simulink model "threePhaseInverterOpenLoop"  (R2021a)
settings: Solver=VariableStepAuto  StartTime=0.0  StopTime=.18  RelTol=1e-3
libraries: spsIGBTDiodeLib x12, spsTHDLib x6, spsSeriesRLCBranchLib x6, spsVoltageMeasurementLib x6, spsDCVoltageSourceLib x4, spsGroundLib x4, spsTriangleGeneratorLib x2, spsCurrentMeasurementLib x2, spspowerguiLib x1
settings Model: Creator=User  LastModifiedBy=User
settings SolverCC: AlgebraicLoopSolver=TrustRegion
settings DebuggingCC: SFMachineParentedDataDiag=warning

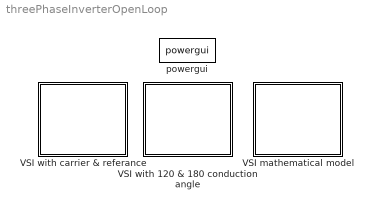
== system threePhaseInverterOpenLoop ==
  VSI mathematical model : Subsystem
  VSI with 120 & 180 conduction angle : Subsystem
  VSI with carrier & referance : Subsystem
  powergui : spspowerguiLib/powergui  Priority=1  SimulationMode=Continuous  SampleTime=50e-6  frequency=60  Iterations=50  frequencyindice=0  Pbase=100e6  ErrMax=1e-4  UnitsV=kV  UnitsW=MW  buscounter=0  FunctionMessages=off  echomessages=off  EnableUseOfTLC=off  CurrentSourceSwitches=off  DisableSnubberDevices=on  DisableRonSwitches=on  DisableVfSwitches=on  DisplayEquations=off  AutomaticDiscreteSolvers=off  SolverType=Tustin/Backward Euler (TBE)  Interpol=off  ExternalGateDelay=off  methode=off  Ts=100  x0status=blocks  SPID=on  SwTol=0  HookPort=off  NonlinearTolerance=1e-4  nMaxIteration=100  ContinueOnMaxIteration=off  RestoreLinks=warning  ResistiveCurrentMeasurement=off  Frange=[0:2:500]  Ylog=off  Xlog=on  ShowGrid=off  save=off  variable=ZData  structure=0  ZoomFFT=off  StartTime=0.0  cycles=1  DisplayStyle=1  fundamental=60  FreqAxis=off  MaxFrequency=1000  frequencyindicesteady=1  RmsSteady=1  display=off

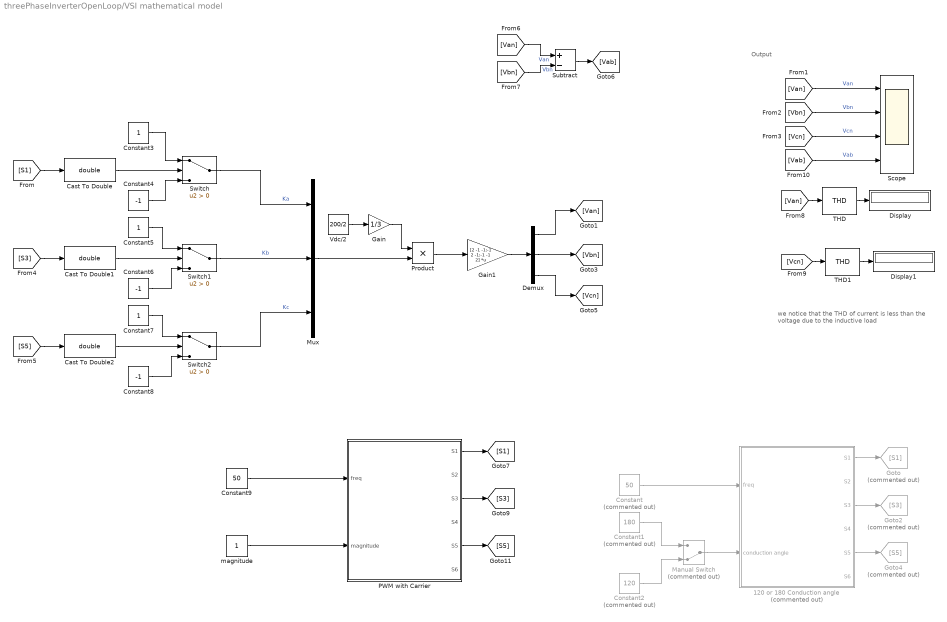
== system threePhaseInverterOpenLoop/VSI mathematical model ==
  note: we notice that the THD of current is less than the voltage due to the inductive load
  note: Output
  120 or 180 Conduction angle : Subsystem  Commented=on
  Cast To Double : DataTypeConversion  OutDataTypeStr=double
  Cast To Double1 : DataTypeConversion  OutDataTypeStr=double
  Cast To Double2 : DataTypeConversion  OutDataTypeStr=double
  Constant : Constant  Commented=on  Value=50
  Constant1 : Constant  Commented=on  Value=180
  Constant2 : Constant  Commented=on  Value=120
  Constant3 : Constant
  Constant4 : Constant  Value=-1
  Constant5 : Constant
  Constant6 : Constant  Value=-1
  Constant7 : Constant
  Constant8 : Constant  Value=-1
  Constant9 : Constant  Value=50
  Demux : Demux  Outputs=3
  Display : Display
  Display1 : Display
  Gain : Gain  Gain=1/3
  Gain1 : Gain  Gain=[2 -1 -1;-1 2 -1;-1 -1 2]  Multiplication=Matrix(K*u)
  Goto : Goto  Commented=on  GotoTag=S1
  Goto2 : Goto  Commented=on  GotoTag=S3
  Goto4 : Goto  Commented=on  GotoTag=S5
  Manual Switch : ManualSwitch  Commented=on  CurrentSetting=0
  Mux : Mux  Inputs=3
  PWM with Carrier : Subsystem
  Product : Product
  Scope : Scope  NumInputPorts=4
  Subtract : Sum  Inputs=+-
  Switch : Switch  Criteria=u2 > Threshold
  Switch1 : Switch  Criteria=u2 > Threshold
  Switch2 : Switch  Criteria=u2 > Threshold
  THD : spsTHDLib/THD  Freq=60  Ts=0
      settings: SourceProductBaseCode=PS
  THD1 : spsTHDLib/THD  Freq=60  Ts=0
      settings: SourceProductBaseCode=PS
  Vdc/2 : Constant  Value=200/2
  magnitude : Constant
  wires:
  Constant1/1 -> Manual Switch/1
  THD1/1 -> Display1/1
  [Van] -> Scope/1  "Van"
  [Vbn] -> Scope/2  "Vbn"
  [Vcn] -> THD1/1
  [Van] -> THD/1
  Constant/1 -> 120 or 180 Conduction angle/1(freq)
  120 or 180 Conduction angle/3(S3) -> Goto2/1
  120 or 180 Conduction angle/5(S5) -> Goto4/1
  THD/1 -> Display/1
  Constant2/1 -> Manual Switch/2
  120 or 180 Conduction angle/1(S1) -> Goto/1
  [Vcn] -> Scope/3  "Vcn"
  Manual Switch/1 -> 120 or 180 Conduction angle/2(conduction angle)
  [S3] -> Cast To Double1/1
  Switch/1 -> Mux/1  "Ka"
  [S5] -> Cast To Double2/1
  Switch1/1 -> Mux/2  "Kb"
  Gain/1 -> Product/1
  Demux/3 -> [Vcn]
  Demux/2 -> [Vbn]
  [S1] -> Cast To Double/1
  Gain1/1 -> Demux/1
  Cast To Double/1 -> Switch/2
  Product/1 -> Gain1/1
  Vdc/2/1 -> Gain/1
  Mux/1 -> Product/2
  Demux/1 -> [Van]
  Constant3/1 -> Switch/1
  Constant4/1 -> Switch/3
  Constant6/1 -> Switch1/3
  Constant5/1 -> Switch1/1
  Cast To Double1/1 -> Switch1/2
  Cast To Double2/1 -> Switch2/2
  Constant7/1 -> Switch2/1
  Constant8/1 -> Switch2/3
  Switch2/1 -> Mux/3  "Kc"
  [Van] -> Subtract/1  "Van"
  [Vbn] -> Subtract/2  "Vbn"
  Subtract/1 -> [Vab]
  [Vab] -> Scope/4  "Vab"
  magnitude/1 -> PWM with Carrier/2(magnitude)
  PWM with Carrier/5(S5) -> [S5]
  Constant9/1 -> PWM with Carrier/1(freq)
  PWM with Carrier/3(S3) -> [S3]
  PWM with Carrier/1(S1) -> [S1]

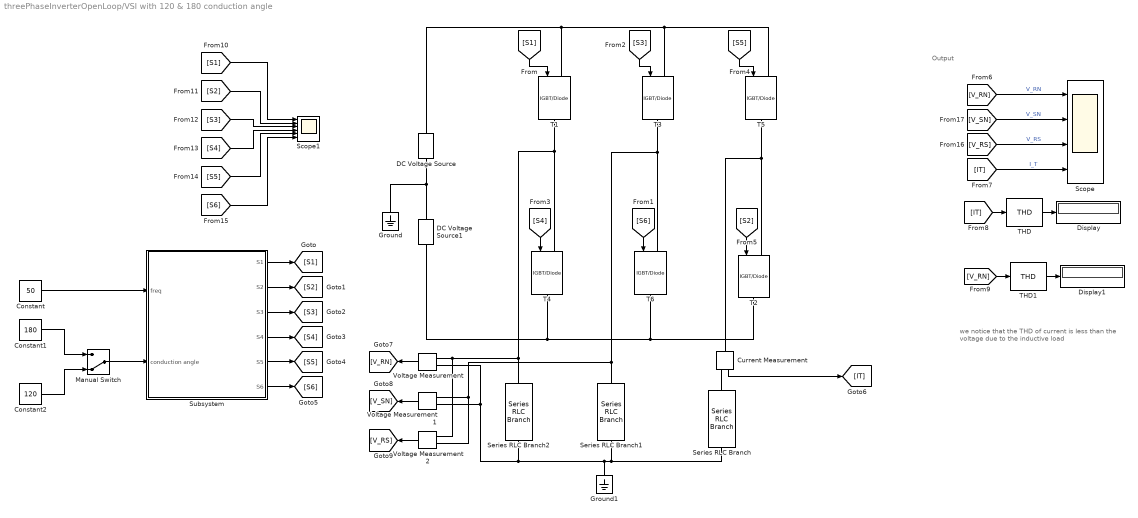
== system threePhaseInverterOpenLoop/VSI with 120 & 180 conduction angle ==
  note: Output
  note: we notice that the THD of current is less than the voltage due to the inductive load
  Constant : Constant  Value=50
  Constant1 : Constant  Value=180
  Constant2 : Constant  Value=120
  Current Measurement : spsCurrentMeasurementLib/Current Measurement  PhasorSimulation=off  OutputType=Complex  PSBequivalent=0
  DC Voltage Source : spsDCVoltageSourceLib/DC Voltage Source  Amplitude=100  Measurements=None
  DC Voltage Source1 : spsDCVoltageSourceLib/DC Voltage Source  Amplitude=100  Measurements=None
  Display : Display
  Display1 : Display
  Ground : spsGroundLib/Ground  LConnTagsString=a
  Ground1 : spsGroundLib/Ground  LConnTagsString=a
  Manual Switch : ManualSwitch  CurrentSetting=0
  Scope : Scope  NumInputPorts=4
  Scope1 : Scope  NumInputPorts=6
  Series RLC Branch : spsSeriesRLCBranchLib/Series RLC Branch  LConnTagsString=__new0  RConnTagsString=__new0  BranchType=R  Resistance=10  Inductance=50e-3  SetiL0=off  InitialCurrent=0  Capacitance=1e-6  Setx0=off  InitialVoltage=0  Measurements=None
  Series RLC Branch1 : spsSeriesRLCBranchLib/Series RLC Branch  LConnTagsString=__new0  RConnTagsString=__new0  BranchType=R  Resistance=10  Inductance=50e-3  SetiL0=off  InitialCurrent=0  Capacitance=1e-6  Setx0=off  InitialVoltage=0  Measurements=None
  Series RLC Branch2 : spsSeriesRLCBranchLib/Series RLC Branch  LConnTagsString=__new0  RConnTagsString=__new0  BranchType=R  Resistance=10  Inductance=50e-3  SetiL0=off  InitialCurrent=0  Capacitance=1e-6  Setx0=off  InitialVoltage=0  Measurements=None
  Subsystem : Subsystem
  T{1..6} (6 alike) : spsIGBTDiodeLib/IGBT//Diode  Ron=1e-3  Rs=1e5  Cs=inf  Measurements=off
  THD : spsTHDLib/THD  Freq=60  Ts=0
      settings: SourceProductBaseCode=PS
  THD1 : spsTHDLib/THD  Freq=60  Ts=0
      settings: SourceProductBaseCode=PS
  Voltage Measurement : spsVoltageMeasurementLib/Voltage Measurement  PhasorSimulation=off  OutputType=Complex  PSBequivalent=0
  Voltage Measurement1 : spsVoltageMeasurementLib/Voltage Measurement  PhasorSimulation=off  OutputType=Complex  PSBequivalent=0
  Voltage Measurement2 : spsVoltageMeasurementLib/Voltage Measurement  PhasorSimulation=off  OutputType=Complex  PSBequivalent=0
  wires:
  Manual Switch/1 -> Subsystem/2(conduction angle)
  Voltage Measurement1/1 -> [V_SN]
  [S2] -> Scope1/2
  [V_RS] -> Scope/3  "V_RS"
  Voltage Measurement2/1 -> [V_RS]
  Subsystem/1(S1) -> [S1]
  Constant2/1 -> Manual Switch/2
  Current Measurement/1 -> [IT]
  THD/1 -> Display/1
  Subsystem/5(S5) -> [S5]
  [S2] -> T2/1
  [S5] -> T5/1
  [S1] -> T1/1
  [S1] -> Scope1/1
  Subsystem/3(S3) -> [S3]
  [S6] -> T6/1
  [S6] -> Scope1/6
  Constant/1 -> Subsystem/1(freq)
  [IT] -> THD/1
  Voltage Measurement/1 -> [V_RN]
  [S4] -> T4/1
  [V_RN] -> THD1/1
  [V_SN] -> Scope/2  "V_SN"
  [IT] -> Scope/4  "I_T"
  [S5] -> Scope1/5
  [S3] -> T3/1
  [V_RN] -> Scope/1  "V_RN"
  [S4] -> Scope1/4
  THD1/1 -> Display1/1
  Subsystem/2(S2) -> [S2]
  Subsystem/6(S6) -> [S6]
  [S3] -> Scope1/3
  Subsystem/4(S4) -> [S4]
  Constant1/1 -> Manual Switch/1
  connections:
  T1/LConn1 -- DC Voltage Source/RConn1 -- T5/LConn1 -- T3/LConn1
  Series RLC Branch/RConn1 -- Series RLC Branch1/RConn1 -- Series RLC Branch2/RConn1 -- Voltage Measurement1/LConn2 -- Voltage Measurement/LConn2 -- Ground1/LConn1
  T3/RConn1 -- Series RLC Branch1/LConn1 -- Voltage Measurement1/LConn1 -- Voltage Measurement2/LConn2 -- T6/LConn1
  DC Voltage Source1/RConn1 -- Ground/LConn1 -- DC Voltage Source/LConn1
  T1/RConn1 -- Voltage Measurement2/LConn1 -- Voltage Measurement/LConn1 -- Series RLC Branch2/LConn1 -- T4/LConn1
  T4/RConn1 -- T2/RConn1 -- T6/RConn1 -- DC Voltage Source1/LConn1
  Series RLC Branch/LConn1 -- Current Measurement/RConn1
  T2/LConn1 -- Current Measurement/LConn1 -- T5/RConn1

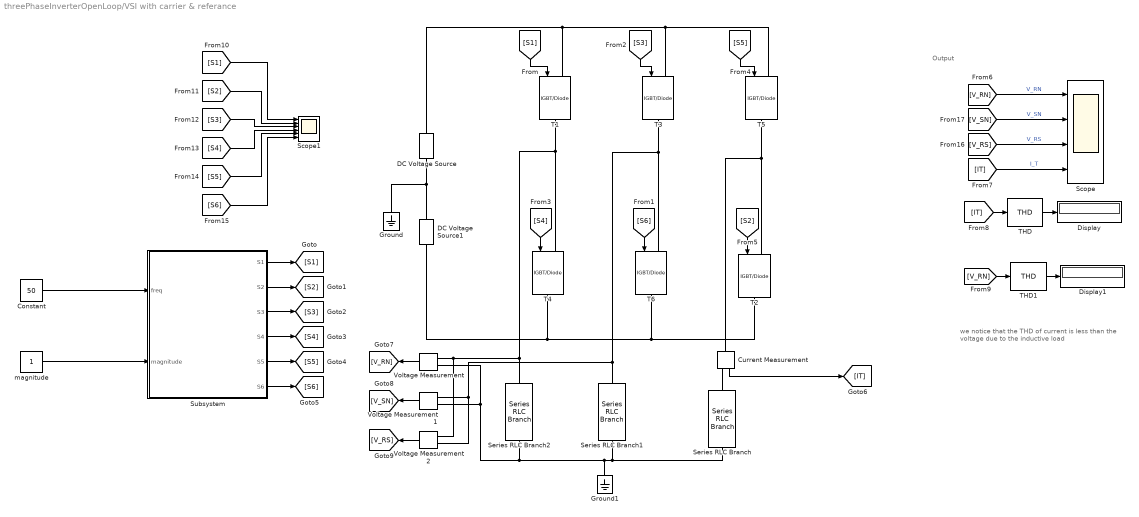
== system threePhaseInverterOpenLoop/VSI with carrier & referance ==
  note: we notice that the THD of current is less than the voltage due to the inductive load
  note: Output
  Constant : Constant  Value=50
  Current Measurement : spsCurrentMeasurementLib/Current Measurement  PhasorSimulation=off  OutputType=Complex  PSBequivalent=0
  DC Voltage Source : spsDCVoltageSourceLib/DC Voltage Source  Amplitude=100  Measurements=None
  DC Voltage Source1 : spsDCVoltageSourceLib/DC Voltage Source  Amplitude=100  Measurements=None
  Display : Display
  Display1 : Display
  Ground : spsGroundLib/Ground  LConnTagsString=a
  Ground1 : spsGroundLib/Ground  LConnTagsString=a
  Scope : Scope  NumInputPorts=4
  Scope1 : Scope  NumInputPorts=6
  Series RLC Branch : spsSeriesRLCBranchLib/Series RLC Branch  LConnTagsString=__new0  RConnTagsString=__new0  BranchType=RL  Resistance=10  Inductance=50e-3  SetiL0=off  InitialCurrent=0  Capacitance=1e-6  Setx0=off  InitialVoltage=0  Measurements=None
  Series RLC Branch1 : spsSeriesRLCBranchLib/Series RLC Branch  LConnTagsString=__new0  RConnTagsString=__new0  BranchType=RL  Resistance=10  Inductance=50e-3  SetiL0=off  InitialCurrent=0  Capacitance=1e-6  Setx0=off  InitialVoltage=0  Measurements=None
  Series RLC Branch2 : spsSeriesRLCBranchLib/Series RLC Branch  LConnTagsString=__new0  RConnTagsString=__new0  BranchType=RL  Resistance=10  Inductance=50e-3  SetiL0=off  InitialCurrent=0  Capacitance=1e-6  Setx0=off  InitialVoltage=0  Measurements=None
  Subsystem : Subsystem
  T{1..6} (6 alike) : spsIGBTDiodeLib/IGBT//Diode  Ron=1e-3  Rs=1e5  Cs=inf  Measurements=off
  THD : spsTHDLib/THD  Freq=60  Ts=0
      settings: SourceProductBaseCode=PS
  THD1 : spsTHDLib/THD  Freq=60  Ts=0
      settings: SourceProductBaseCode=PS
  Voltage Measurement : spsVoltageMeasurementLib/Voltage Measurement  PhasorSimulation=off  OutputType=Complex  PSBequivalent=0
  Voltage Measurement1 : spsVoltageMeasurementLib/Voltage Measurement  PhasorSimulation=off  OutputType=Complex  PSBequivalent=0
  Voltage Measurement2 : spsVoltageMeasurementLib/Voltage Measurement  PhasorSimulation=off  OutputType=Complex  PSBequivalent=0
  magnitude : Constant
  wires:
  Subsystem/4(S4) -> [S4]
  [S3] -> Scope1/3
  Subsystem/6(S6) -> [S6]
  Subsystem/2(S2) -> [S2]
  THD1/1 -> Display1/1
  [S4] -> Scope1/4
  [V_RN] -> Scope/1  "V_RN"
  [S3] -> T3/1
  [S5] -> Scope1/5
  [IT] -> Scope/4  "I_T"
  [V_SN] -> Scope/2  "V_SN"
  [V_RN] -> THD1/1
  [S4] -> T4/1
  Voltage Measurement/1 -> [V_RN]
  [IT] -> THD/1
  Constant/1 -> Subsystem/1(freq)
  [S6] -> Scope1/6
  [S6] -> T6/1
  Subsystem/3(S3) -> [S3]
  [S1] -> Scope1/1
  [S1] -> T1/1
  [S5] -> T5/1
  [S2] -> T2/1
  Subsystem/5(S5) -> [S5]
  THD/1 -> Display/1
  Current Measurement/1 -> [IT]
  Subsystem/1(S1) -> [S1]
  Voltage Measurement2/1 -> [V_RS]
  [V_RS] -> Scope/3  "V_RS"
  [S2] -> Scope1/2
  Voltage Measurement1/1 -> [V_SN]
  magnitude/1 -> Subsystem/2(magnitude)
  connections:
  T5/RConn1 -- Current Measurement/LConn1 -- T2/LConn1
  Series RLC Branch/LConn1 -- Current Measurement/RConn1
  DC Voltage Source1/LConn1 -- T4/RConn1 -- T6/RConn1 -- T2/RConn1
  Series RLC Branch2/LConn1 -- Voltage Measurement/LConn1 -- Voltage Measurement2/LConn1 -- T4/LConn1 -- T1/RConn1
  DC Voltage Source/LConn1 -- Ground/LConn1 -- DC Voltage Source1/RConn1
  T6/LConn1 -- T3/RConn1 -- Voltage Measurement2/LConn2 -- Voltage Measurement1/LConn1 -- Series RLC Branch1/LConn1
  Series RLC Branch1/RConn1 -- Series RLC Branch/RConn1 -- Ground1/LConn1 -- Voltage Measurement/LConn2 -- Voltage Measurement1/LConn2 -- Series RLC Branch2/RConn1
  T3/LConn1 -- T5/LConn1 -- T1/LConn1 -- DC Voltage Source/RConn1

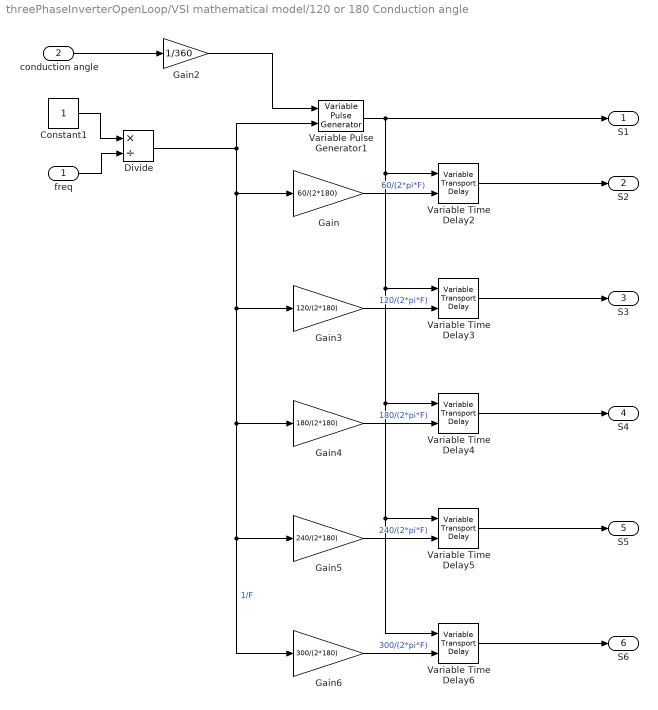
== system threePhaseInverterOpenLoop/VSI mathematical model/120 or 180 Conduction angle ==
  freq : Inport
  conduction angle : Inport  Port=2
  Constant1 : Constant
  Divide : Product  Inputs=*/
  Gain : Gain  Gain=60/(2*180)
  Gain2 : Gain  Gain=1/360
  Gain3 : Gain  Gain=120/(2*180)
  Gain4 : Gain  Gain=180/(2*180)
  Gain5 : Gain  Gain=240/(2*180)
  Gain6 : Gain  Gain=300/(2*180)
  Variable Time Delay{2..6} (5 alike) : VariableTransportDelay  MaximumDelay=10
  Variable Pulse Generator1 : VariablePulseGenerator  RunAtFixedTimeIntervals=on  SampleTime=.00001
  S1 : Outport
  S2 : Outport  Port=2
  S3 : Outport  Port=3
  S4 : Outport  Port=4
  S5 : Outport  Port=5
  S6 : Outport  Port=6
  wires:
  Gain6/1 -> Variable Time Delay6/2  "300/(2*pi*F)"
  Gain5/1 -> Variable Time Delay5/2  "240/(2*pi*F)"
  Gain4/1 -> Variable Time Delay4/2  "180/(2*pi*F)"
  Gain3/1 -> Variable Time Delay3/2  "120/(2*pi*F)"
  Gain/1 -> Variable Time Delay2/2  "60/(2*pi*F)"
  Divide/1 -> Gain/1, Gain4/1, Gain6/1, Gain5/1, Gain3/1, Variable Pulse Generator1/2  "1/F"
  conduction angle/1 -> Gain2/1
  Variable Time Delay6/1 -> S6/1
  Variable Time Delay5/1 -> S5/1
  Variable Time Delay4/1 -> S4/1
  Variable Time Delay3/1 -> S3/1
  Variable Time Delay2/1 -> S2/1
  Variable Pulse Generator1/1 -> Variable Time Delay6/1, Variable Time Delay5/1, Variable Time Delay4/1, Variable Time Delay3/1, Variable Time Delay2/1, S1/1
  Gain2/1 -> Variable Pulse Generator1/1
  Constant1/1 -> Divide/1
  freq/1 -> Divide/2

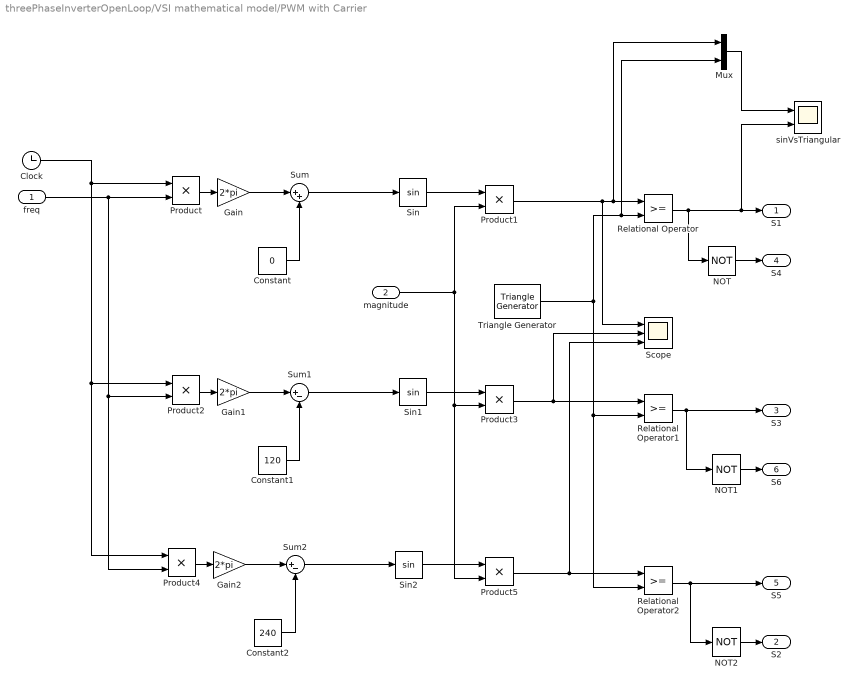
== system threePhaseInverterOpenLoop/VSI mathematical model/PWM with Carrier ==
  freq : Inport
  magnitude : Inport  Port=2
  Clock : Clock
  Constant : Constant  Value=0
  Constant1 : Constant  Value=120
  Constant2 : Constant  Value=240
  Gain : Gain  Gain=2*pi
  Gain1 : Gain  Gain=2*pi
  Gain2 : Gain  Gain=2*pi
  Mux : Mux  Inputs=2
  NOT : Logic  Operator=NOT  IconShape=distinctive  AllPortsSameDT=off  OutDataTypeStr=boolean
  NOT1 : Logic  Operator=NOT  IconShape=distinctive  AllPortsSameDT=off  OutDataTypeStr=boolean
  NOT2 : Logic  Operator=NOT  IconShape=distinctive  AllPortsSameDT=off  OutDataTypeStr=boolean
  Product{,1..5} (6 alike) : Product
  Relational Operator : RelationalOperator  OutDataTypeStr=boolean  RndMeth=Simplest
  Relational Operator1 : RelationalOperator  OutDataTypeStr=boolean  RndMeth=Simplest
  Relational Operator2 : RelationalOperator  OutDataTypeStr=boolean  RndMeth=Simplest
  Scope : Scope  NumInputPorts=3
  Sin : Trigonometry
  Sin1 : Trigonometry
  Sin2 : Trigonometry
  Sum : Sum  Inputs=|++
  Sum1 : Sum  Inputs=|+-
  Sum2 : Sum  Inputs=|+-
  Triangle Generator : spsTriangleGeneratorLib/Triangle Generator  Freq=5e3  Phase=90  Ts=0
  sinVsTriangular : Scope  NumInputPorts=2
  S1 : Outport
  S2 : Outport  Port=2
  S3 : Outport  Port=3
  S4 : Outport  Port=4
  S5 : Outport  Port=5
  S6 : Outport  Port=6
  wires:
  Sum/1 -> Sin/1
  Constant/1 -> Sum/2
  Product/1 -> Gain/1
  Gain/1 -> Sum/1
  Sin/1 -> Product1/1
  Sin1/1 -> Product3/1
  Gain1/1 -> Sum1/1
  Product2/1 -> Gain1/1
  Constant1/1 -> Sum1/2
  Sum1/1 -> Sin1/1
  Sum2/1 -> Sin2/1
  Constant2/1 -> Sum2/2
  Product4/1 -> Gain2/1
  Clock/1 -> Product/1, Product2/1, Product4/1
  freq/1 -> Product2/2, Product4/2, Product/2
  Gain2/1 -> Sum2/1
  Sin2/1 -> Product5/1
  magnitude/1 -> Product5/2, Product3/2, Product1/2
  Product1/1 -> Scope/1, Mux/1, Relational Operator/1
  Product3/1 -> Scope/2, Relational Operator1/1
  Product5/1 -> Scope/3, Relational Operator2/1
  Triangle Generator/1 -> Relational Operator2/2, Relational Operator1/2, Mux/2, Relational Operator/2
  Relational Operator/1 -> NOT/1, sinVsTriangular/2, S1/1
  NOT/1 -> S4/1
  Relational Operator1/1 -> NOT1/1, S3/1
  NOT1/1 -> S6/1
  Relational Operator2/1 -> NOT2/1, S5/1
  NOT2/1 -> S2/1
  Mux/1 -> sinVsTriangular/1

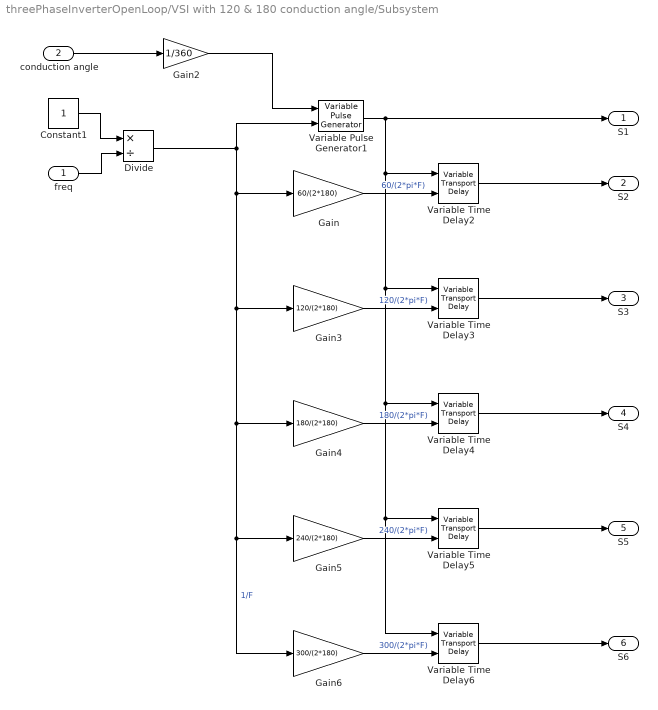
== system threePhaseInverterOpenLoop/VSI with 120 & 180 conduction angle/Subsystem ==
  freq : Inport
  conduction angle : Inport  Port=2
  Constant1 : Constant
  Divide : Product  Inputs=*/
  Gain : Gain  Gain=60/(2*180)
  Gain2 : Gain  Gain=1/360
  Gain3 : Gain  Gain=120/(2*180)
  Gain4 : Gain  Gain=180/(2*180)
  Gain5 : Gain  Gain=240/(2*180)
  Gain6 : Gain  Gain=300/(2*180)
  Variable Time Delay{2..6} (5 alike) : VariableTransportDelay  MaximumDelay=10
  Variable Pulse Generator1 : VariablePulseGenerator  RunAtFixedTimeIntervals=on  SampleTime=.00001
  S1 : Outport
  S2 : Outport  Port=2
  S3 : Outport  Port=3
  S4 : Outport  Port=4
  S5 : Outport  Port=5
  S6 : Outport  Port=6
  wires:
  freq/1 -> Divide/2
  Constant1/1 -> Divide/1
  Gain2/1 -> Variable Pulse Generator1/1
  Variable Pulse Generator1/1 -> S1/1, Variable Time Delay2/1, Variable Time Delay3/1, Variable Time Delay4/1, Variable Time Delay5/1, Variable Time Delay6/1
  Variable Time Delay2/1 -> S2/1
  Variable Time Delay3/1 -> S3/1
  Variable Time Delay4/1 -> S4/1
  Variable Time Delay5/1 -> S5/1
  Variable Time Delay6/1 -> S6/1
  conduction angle/1 -> Gain2/1
  Divide/1 -> Variable Pulse Generator1/2, Gain3/1, Gain5/1, Gain6/1, Gain4/1, Gain/1  "1/F"
  Gain/1 -> Variable Time Delay2/2  "60/(2*pi*F)"
  Gain3/1 -> Variable Time Delay3/2  "120/(2*pi*F)"
  Gain4/1 -> Variable Time Delay4/2  "180/(2*pi*F)"
  Gain5/1 -> Variable Time Delay5/2  "240/(2*pi*F)"
  Gain6/1 -> Variable Time Delay6/2  "300/(2*pi*F)"

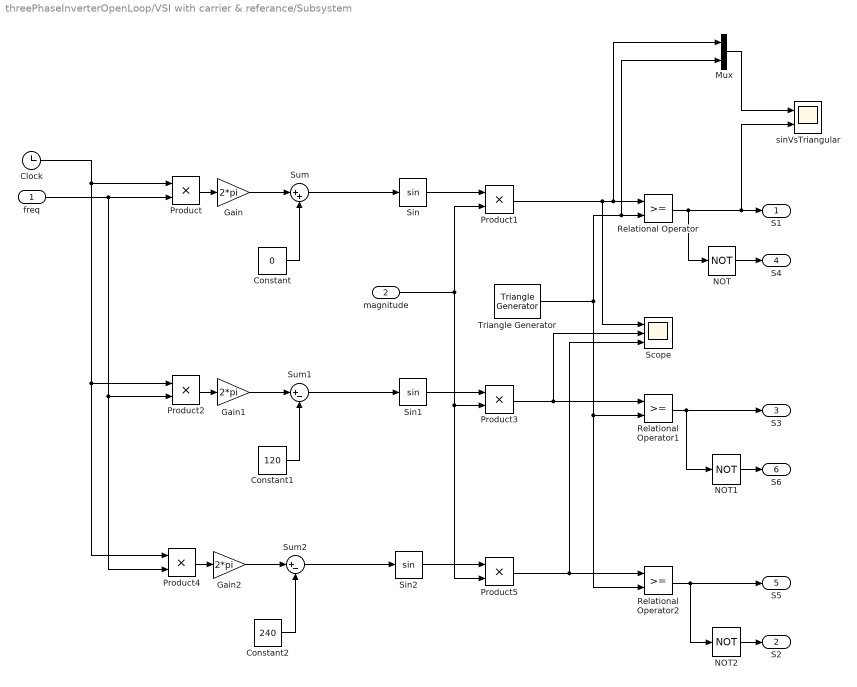
== system threePhaseInverterOpenLoop/VSI with carrier & referance/Subsystem ==
  freq : Inport
  magnitude : Inport  Port=2
  Clock : Clock
  Constant : Constant  Value=0
  Constant1 : Constant  Value=120
  Constant2 : Constant  Value=240
  Gain : Gain  Gain=2*pi
  Gain1 : Gain  Gain=2*pi
  Gain2 : Gain  Gain=2*pi
  Mux : Mux  Inputs=2
  NOT : Logic  Operator=NOT  IconShape=distinctive  AllPortsSameDT=off  OutDataTypeStr=boolean
  NOT1 : Logic  Operator=NOT  IconShape=distinctive  AllPortsSameDT=off  OutDataTypeStr=boolean
  NOT2 : Logic  Operator=NOT  IconShape=distinctive  AllPortsSameDT=off  OutDataTypeStr=boolean
  Product{,1..5} (6 alike) : Product
  Relational Operator : RelationalOperator  OutDataTypeStr=boolean  RndMeth=Simplest
  Relational Operator1 : RelationalOperator  OutDataTypeStr=boolean  RndMeth=Simplest
  Relational Operator2 : RelationalOperator  OutDataTypeStr=boolean  RndMeth=Simplest
  Scope : Scope  NumInputPorts=3
  Sin : Trigonometry
  Sin1 : Trigonometry
  Sin2 : Trigonometry
  Sum : Sum  Inputs=|++
  Sum1 : Sum  Inputs=|+-
  Sum2 : Sum  Inputs=|+-
  Triangle Generator : spsTriangleGeneratorLib/Triangle Generator  Freq=5e3  Phase=90  Ts=0
  sinVsTriangular : Scope  NumInputPorts=2
  S1 : Outport
  S2 : Outport  Port=2
  S3 : Outport  Port=3
  S4 : Outport  Port=4
  S5 : Outport  Port=5
  S6 : Outport  Port=6
  wires:
  Sum/1 -> Sin/1
  Constant/1 -> Sum/2
  Product/1 -> Gain/1
  Gain/1 -> Sum/1
  Sin/1 -> Product1/1
  Sin1/1 -> Product3/1
  Gain1/1 -> Sum1/1
  Product2/1 -> Gain1/1
  Constant1/1 -> Sum1/2
  Sum1/1 -> Sin1/1
  Sum2/1 -> Sin2/1
  Constant2/1 -> Sum2/2
  Product4/1 -> Gain2/1
  Clock/1 -> Product/1, Product2/1, Product4/1
  freq/1 -> Product2/2, Product4/2, Product/2
  Gain2/1 -> Sum2/1
  Sin2/1 -> Product5/1
  magnitude/1 -> Product5/2, Product3/2, Product1/2
  Product1/1 -> Scope/1, Mux/1, Relational Operator/1
  Product3/1 -> Scope/2, Relational Operator1/1
  Product5/1 -> Scope/3, Relational Operator2/1
  Triangle Generator/1 -> Relational Operator2/2, Relational Operator1/2, Mux/2, Relational Operator/2
  Relational Operator/1 -> NOT/1, sinVsTriangular/2, S1/1
  NOT/1 -> S4/1
  Relational Operator1/1 -> NOT1/1, S3/1
  NOT1/1 -> S6/1
  Relational Operator2/1 -> NOT2/1, S5/1
  NOT2/1 -> S2/1
  Mux/1 -> sinVsTriangular/1
